simulink model "exampleMinStopTime"  (R2016b)
settings: Solver=ode45  StartTime=0.0  StopTime=30  RelTol=1e-3  EnableMultiTasking=on
libraries: carnot x2
settings Model: Creator=drhf  LastModifiedBy=drhf
settings DataIOCC: LimitDataPoints=on  SaveFormat=Array  SignalLoggingSaveFormat=ModelDataLogs
settings OptimizationCC: ExpressionDepthLimit=2147483647  LifeSpan=inf
settings DebuggingCC: UnderspecifiedInitializationDetection=Classic  MergeDetectMultiDrivingBlocksExec=none  SolverPrmCheckMsg=warning  StateNameClashWarn=warning  SFUnexpectedBacktrackingDiag=warning  SFNoUnconditionalDefaultTransitionDiag=warning  SFExecutionAtInitializationDiag=none
settings HardwareCC: ProdBitPerPointer=32  ProdBitPerSizeT=32  ProdBitPerPtrDiffT=32  ProdLargestAtomicFloat=None  ProdIntDivRoundTo=Undefined  ProdEndianess=Unspecified  ProdWordSize=32  ProdHWDeviceType=32-bit Generic
settings ModelReferenceCC: PropagateSignalLabelsOutOfModel=off
settings GRTTargetCC: TargetLangStandard=C89/C90 (ANSI)  GeneratePreprocessorConditionals=Disable all  CombineOutputUpdateFcns=off  GRTInterface=on
settings ConfigComp: CovMetricSettings=dw  CovHtmlReporting=on  CovSaveCumulativeToWorkspaceVar=on  CovSaveSingleToWorkspaceVar=on  CovExternalEMLEnable=off

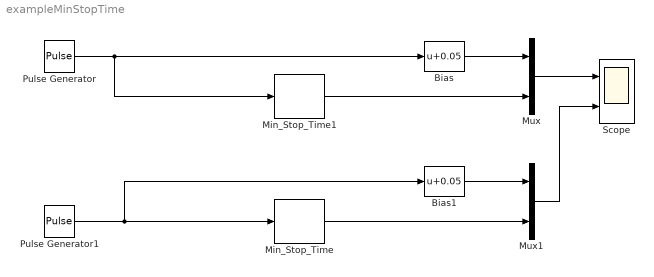
== system exampleMinStopTime ==
  Bias : Bias  Bias=0.05
  Bias1 : Bias  Bias=0.05
  Min_Stop_Time : carnot/Control/Min_Stop_Time  tminstop=15
  Min_Stop_Time1 : carnot/Control/Min_Stop_Time  tminstop=15
  Mux : Mux  Inputs=2
  Mux1 : Mux  Inputs=2
  Pulse Generator : DiscretePulseGenerator  PulseType=Time based  Amplitude=2  Period=10  PulseWidth=80
  Pulse Generator1 : DiscretePulseGenerator  PulseType=Time based  Amplitude=2  Period=8  PulseWidth=5
  Scope : Scope  NumInputPorts=2
  wires:
  Pulse Generator/1 -> Bias/1, Min_Stop_Time1/1
  Mux/1 -> Scope/1
  Min_Stop_Time1/1 -> Mux/2
  Pulse Generator1/1 -> Bias1/1, Min_Stop_Time/1
  Min_Stop_Time/1 -> Mux1/2
  Mux1/1 -> Scope/2
  Bias/1 -> Mux/1
  Bias1/1 -> Mux1/1
